simulink model "gm_Transformation_V12"  (R2018a)
settings: Solver=FixedStepDiscrete  StartTime=0.0  StopTime=10.0  RelTol=1e-3
InitFcn:
  | Ts_xadc = 0.1;
undefined symbols (not defined in the file or in its folder): T_25MHz, T_mech
libraries: hdlsllib x14, simulink x12, hdlmdlgenlib x5, simulink_need_slupdate x1
(part 2 of 4)

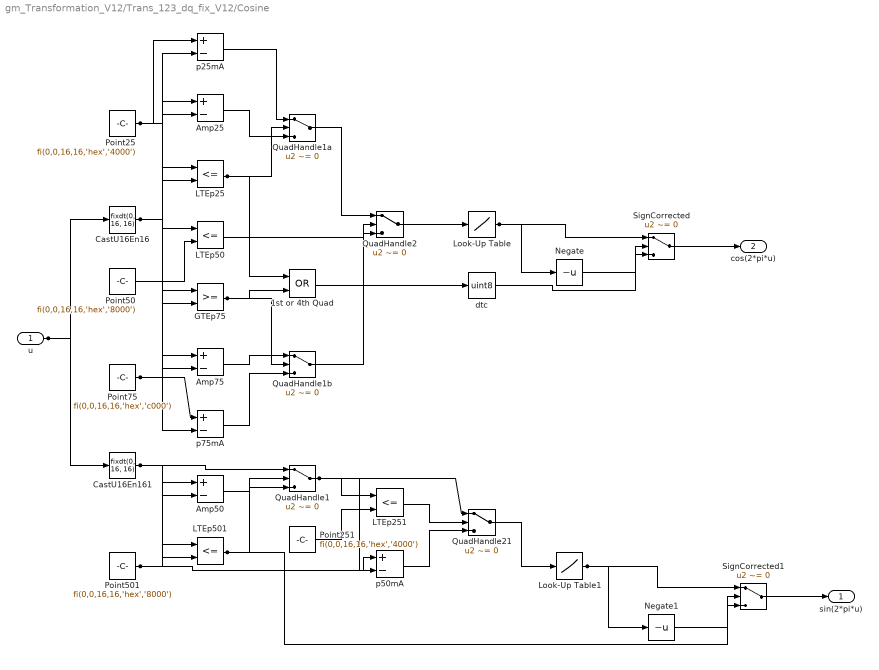
== system gm_Transformation_V12/Trans_123_dq_fix_V12/Cosine ==
  u : Inport  OutDataTypeStr=fixdt(1, 24, 20)  SampleTime=4e-08
  1st or 4th Quad : Logic  Operator=OR  AllPortsSameDT=off  OutDataTypeStr=boolean  SampleTime=4e-08
  Amp25 : Sum  Inputs=+-  AccumDataTypeStr=fixdt(1, 17, 16)  OutDataTypeStr=fixdt(1, 17, 16)  SampleTime=4e-08
  Amp50 : Sum  Inputs=+-  AccumDataTypeStr=fixdt(1, 17, 16)  OutDataTypeStr=fixdt(1, 17, 16)  SampleTime=4e-08
  Amp75 : Sum  Inputs=+-  AccumDataTypeStr=fixdt(1, 17, 16)  OutDataTypeStr=fixdt(1, 17, 16)  SampleTime=4e-08
  CastU16En16 : DataTypeConversion  OutDataTypeStr=fixdt(0, 16, 16)  SampleTime=4e-08
  CastU16En161 : DataTypeConversion  OutDataTypeStr=fixdt(0, 16, 16)  SampleTime=4e-08
  GTEp75 : RelationalOperator  OutDataTypeStr=boolean  SampleTime=4e-08  RndMeth=Nearest
  LTEp{25,50,251,501} (4 alike) : RelationalOperator  Operator=<=  OutDataTypeStr=boolean  SampleTime=4e-08  RndMeth=Nearest
  Look-Up Table : Lookup_n-D  NumberOfTableDimensions=1  BreakpointsForDimension1=[0 0.00048828125 0.0009765625 0.00146484375 0.001953125 0.00244140625 0.0029296875 0.00341796875 0.00390625 0.00439453125 0.0048828125 0.00537109375 0.005859375 0.00634765625 0.0068359375 0.00732421875 0.0078125 0.00830078125 0.0087890625 0.00927734375 0.009765625 0.01025390625 0.0107421875 0.01123046875 0.01171875 0.01220703125 0.0126953125 0.01318359375 0.013671875 0.01416015625 0.0146484375 0.01513671875 0.015625 0.01611328125 0.0166015625 0.01708984375 0.017578125 0.01806640625 0.0185546875 0.01904296875 0.01953125 0.02001953125 0.0205078125 0.02099609375 0.021484375 0.02197265625 0.0224609375 0.02294921875 0.0234375 0.02392578125 0.0244140625 0.02490234375 0.025390625 0.02587890625 0.0263671875 0.02685546875 0.02734375 0.02783203125 0.0283203125 0.02880859375 0.029296875 0.02978515625 0.0302734375 0.03076171875 0.03125 0.03173828125 0.0322265625 0.03271484375 0.033203125 0.03369140625 0.0341796875 0.03466796875 0.03515625 0.03564453125 0.0361328125 0.03662109375 0.037109375 0.03759765625 0.0380859375 0.03857421875 0.0390625 0.03955078125 0.0400390625 0.04052734375 0.041015625 0.04150390625 0.0419921875 0.04248046875 0.04296875 0.04345703125 0.0439453125 0.04443359375 0.044921875 0.04541015625 0.0458984375 0.04638671875 0.046875 0.04736328125 0.0478515625 0.04833984375 0.048828125 0.04931640625 0.0498046875 0.05029296875 0.05078125 0.05126953125 0.0517578125 0.05224609375 0.052734375 0.05322265625 0.0537109375 0.05419921875 0.0546875 0.05517578125 0.0556640625 0.05615234375 0.056640625 0.05712890625 0.0576171875 0.05810546875 0.05859375 0.05908203125 0.0595703125 0.06005859375 0.060546875 0.06103515625 0.0615234375 0.06201171875 0.0625 0.06298828125 0.0634765625 0.06396484375 0.064453125 0.06494140625 0.0654296875 0.06591796875 0.06640625 0.06689453125 0.0673828125 0.06787109375 0.068359375 0.06884765625 0.0693359375 0.06982421875 0.0703125 0.07080078125 0.0712890625 0.07177734375 0.072265625 0.07275390625 0.0732421875 0.07373046875 0.07421875 0.07470703125 0.0751953125 0.07568359375 0.076171875 0.07666015625 0.0771484375 0.07763671875 0.078125 0.07861328125 0.0791015625 0.07958984375 0.080078125 0.08056640625 0.0810546875 0.08154296875 0.08203125 0.08251953125 0.0830078125 0.08349609375 0.083984375 0.08447265625 0.0849609375 0.08544921875 0.0859375 0.08642578125 0.0869140625 0.08740234375 0.087890625 0.08837890625 0.0888671875 0.08935546875 0.08984375 0.09033203125 0.0908203125 0.09130859375 0.091796875 0.09228515625 0.0927734375 0.09326171875 0.09375 0.09423828125 0.0947265625 0.09521484375 0.095703125 0.09619140625 0.0966796875 0.09716796875 0.09765625 0.09814453125 0.0986328125 0.09912109375 0.099609375 0.10009765625 0.1005859375 0.10107421875 0.1015625 0.10205078125 0.1025390625 0.10302734375 0.103515625 0.10400390625 0.1044921875 0.10498046875 0.10546875 0.10595703125 0.1064453125 0.10693359375 0.107421875 0.10791015625 0.1083984375 0.10888671875 0.109375 0.10986328125 0.1103515625 0.11083984375 0.111328125 0.11181640625 0.1123046875 0.11279296875 0.11328125 0.11376953125 0.1142578125 0.11474609375 0.115234375 0.11572265625 0.1162109375 0.11669921875 0.1171875 0.11767578125 0.1181640625 0.11865234375 0.119140625 0.11962890625 0.1201171875 0.12060546875 0.12109375 0.12158203125 0.1220703125 0.12255859375 0.123046875 0.12353515625 0.1240234375 0.12451171875 0.125 0.12548828125 0.1259765625 0.12646484375 0.126953125 0.12744140625 0.1279296875 0.12841796875 0.12890625 0.12939453125 0.1298828125 0.13037109375 0.130859375 0.13134765625 0.1318359375 0.13232421875 0.1328125 0.13330078125 0.1337890625 0.13427734375 0.134765625 0.13525390625 0.1357421875 0.13623046875 0.13671875 0.13720703125 0.1376953125 0.13818359375 0.138671875 0.13916015625 0.1396484375 0.14013671875 0.140625 0.14111328125 0.1416015625 0.14208984375 0.142578125 0.14306640625 0.1435546875 0.14404296875 0.14453125 0.14501953125 0.1455078125 0.14599609375 0.146484375 0.14697265625 0.1474609375 0.14794921875 0.1484375 0.14892578125 0.1494140625 0.14990234375 ...(+2661 chars)]  Table="reshape([0;0.0030517578125;0.00616455078125;0.00921630859375;0.01226806640625;0.01531982421875;0.0184326171875;0.021484375;0.0245361328125;0.027587890625;0.03070068359375;0.03375244140625;0.03680419921875;0.03985595703125;0.04296875;0.0460205078125;0.049072265625;0.0521240234375;0.05517578125;0.05828857421875;0.06134033203125;0.06439208984375;0.06744384765625;0.07049560546875;0.07354736328125;0.07659912109375;0.0797119140625;0.082763671875;0.0858154296875;0.0888671875;0.0919189453125;0.094970703125;0.0980224609375;0.10107421875;0.1041259765625;0.107177734375;0.1102294921875;0.11328125;0.1163330078125;0.119384765625;0.1224365234375;0.12542724609375;0.12847900390625;0.13153076171875;0.13458251953125;0.13763427734375;0.14068603515625;0.1436767578125;0.146728515625;0.1497802734375;0.15277099609375;0.15582275390625;0.15887451171875;0.161865234375;0.1649169921875;0.16796875;0.17095947265625;0.17401123046875;0.177001953125;0.17999267578125;0.18304443359375;0.18603515625;0.1890869140625;0.19207763671875;0.195068359375;0.1981201171875;0.20111083984375;0.2041015625;0.20709228515625;0.2100830078125;0.213134765625;0.21612548828125;0.2191162109375;0.22210693359375;0.22509765625;0.22808837890625;0.2310791015625;0.23406982421875;0.23699951171875;0.239990234375;0.24298095703125;0.2459716796875;0.2489013671875;0.25189208984375;0.2548828125;0.2578125;0.26080322265625;0.26373291015625;0.2667236328125;0.2696533203125;0.27264404296875;0.27557373046875;0.27850341796875;0.281494140625;0.284423828125;0.287353515625;0.290283203125;0.293212890625;0.296142578125;0.299072265625;0.302001953125;0.304931640625;0.307861328125;0.310791015625;0.31365966796875;0.31658935546875;0.31951904296875;0.3223876953125;0.3253173828125;0.32818603515625;0.33111572265625;0.333984375;0.3369140625;0.33978271484375;0.3426513671875;0.34552001953125;0.348388671875;0.351318359375;0.35418701171875;0.3570556640625;0.35992431640625;0.36273193359375;0.3656005859375;0.36846923828125;0.371337890625;0.3741455078125;0.37701416015625;0.37982177734375;0.3826904296875;0.385498046875;0.38836669921875;0.39117431640625;0.39398193359375;0.39678955078125;0.39959716796875;0.40240478515625;0.40521240234375;0.40802001953125;0.41082763671875;0.41363525390625;0.41644287109375;0.419189453125;0.4219970703125;0.4248046875;0.42755126953125;0.4302978515625;0.43310546875;0.43585205078125;0.4385986328125;0.44134521484375;0.444091796875;0.44683837890625;0.4495849609375;0.45233154296875;0.455078125;0.45782470703125;0.46051025390625;0.4632568359375;0.46600341796875;0.46868896484375;0.47137451171875;0.47412109375;0.476806640625;0.4794921875;0.482177734375;0.48486328125;0.487548828125;0.490234375;0.492919921875;0.49554443359375;0.49822998046875;0.50091552734375;0.5035400390625;0.50616455078125;0.50885009765625;0.511474609375;0.51409912109375;0.5167236328125;0.51934814453125;0.52197265625;0.52459716796875;0.5272216796875;0.52978515625;0.53240966796875;0.53497314453125;0.53759765625;0.5401611328125;0.542724609375;0.54534912109375;0.54791259765625;0.55047607421875;0.55303955078125;0.5555419921875;0.55810546875;0.5606689453125;0.56317138671875;0.56573486328125;0.5682373046875;0.57080078125;0.57330322265625;0.5758056640625;0.57830810546875;0.580810546875;0.58331298828125;0.5858154296875;0.5882568359375;0.59075927734375;0.59326171875;0.595703125;0.59814453125;0.60064697265625;0.60308837890625;0.60552978515625;0.60797119140625;0.61041259765625;0.61279296875;0.615234375;0.61767578125;0.62005615234375;0.6224365234375;0.6248779296875;0.62725830078125;0.629638671875;0.63201904296875;0.6343994140625;0.63677978515625;0.63909912109375;0.6414794921875;0.64385986328125;0.64617919921875;0.64849853515625;0.65081787109375;0.6531982421875;0.655517578125;0.6578369140625;0.66009521484375;0.66241455078125;0.66473388671875;0.6669921875;0.6693115234375;0.67156982421875;0.673828125;0.67608642578125;0.6783447265625;0.68060302734375;0.682861328125;0.68505859375;0.68731689453125;0.68951416015625;0.6917724609375;0.6939697265625;0.6961669921875 ...(+4158 chars)])"  ExtrapMethod=Clip  SampleTime=4e-08  OutDataTypeStr=fixdt(1, 16, 14)  InputSameDT=on
  Look-Up Table1 : Lookup_n-D  NumberOfTableDimensions=1  BreakpointsForDimension1=[0 0.00048828125 0.0009765625 0.00146484375 0.001953125 0.00244140625 0.0029296875 0.00341796875 0.00390625 0.00439453125 0.0048828125 0.00537109375 0.005859375 0.00634765625 0.0068359375 0.00732421875 0.0078125 0.00830078125 0.0087890625 0.00927734375 0.009765625 0.01025390625 0.0107421875 0.01123046875 0.01171875 0.01220703125 0.0126953125 0.01318359375 0.013671875 0.01416015625 0.0146484375 0.01513671875 0.015625 0.01611328125 0.0166015625 0.01708984375 0.017578125 0.01806640625 0.0185546875 0.01904296875 0.01953125 0.02001953125 0.0205078125 0.02099609375 0.021484375 0.02197265625 0.0224609375 0.02294921875 0.0234375 0.02392578125 0.0244140625 0.02490234375 0.025390625 0.02587890625 0.0263671875 0.02685546875 0.02734375 0.02783203125 0.0283203125 0.02880859375 0.029296875 0.02978515625 0.0302734375 0.03076171875 0.03125 0.03173828125 0.0322265625 0.03271484375 0.033203125 0.03369140625 0.0341796875 0.03466796875 0.03515625 0.03564453125 0.0361328125 0.03662109375 0.037109375 0.03759765625 0.0380859375 0.03857421875 0.0390625 0.03955078125 0.0400390625 0.04052734375 0.041015625 0.04150390625 0.0419921875 0.04248046875 0.04296875 0.04345703125 0.0439453125 0.04443359375 0.044921875 0.04541015625 0.0458984375 0.04638671875 0.046875 0.04736328125 0.0478515625 0.04833984375 0.048828125 0.04931640625 0.0498046875 0.05029296875 0.05078125 0.05126953125 0.0517578125 0.05224609375 0.052734375 0.05322265625 0.0537109375 0.05419921875 0.0546875 0.05517578125 0.0556640625 0.05615234375 0.056640625 0.05712890625 0.0576171875 0.05810546875 0.05859375 0.05908203125 0.0595703125 0.06005859375 0.060546875 0.06103515625 0.0615234375 0.06201171875 0.0625 0.06298828125 0.0634765625 0.06396484375 0.064453125 0.06494140625 0.0654296875 0.06591796875 0.06640625 0.06689453125 0.0673828125 0.06787109375 0.068359375 0.06884765625 0.0693359375 0.06982421875 0.0703125 0.07080078125 0.0712890625 0.07177734375 0.072265625 0.07275390625 0.0732421875 0.07373046875 0.07421875 0.07470703125 0.0751953125 0.07568359375 0.076171875 0.07666015625 0.0771484375 0.07763671875 0.078125 0.07861328125 0.0791015625 0.07958984375 0.080078125 0.08056640625 0.0810546875 0.08154296875 0.08203125 0.08251953125 0.0830078125 0.08349609375 0.083984375 0.08447265625 0.0849609375 0.08544921875 0.0859375 0.08642578125 0.0869140625 0.08740234375 0.087890625 0.08837890625 0.0888671875 0.08935546875 0.08984375 0.09033203125 0.0908203125 0.09130859375 0.091796875 0.09228515625 0.0927734375 0.09326171875 0.09375 0.09423828125 0.0947265625 0.09521484375 0.095703125 0.09619140625 0.0966796875 0.09716796875 0.09765625 0.09814453125 0.0986328125 0.09912109375 0.099609375 0.10009765625 0.1005859375 0.10107421875 0.1015625 0.10205078125 0.1025390625 0.10302734375 0.103515625 0.10400390625 0.1044921875 0.10498046875 0.10546875 0.10595703125 0.1064453125 0.10693359375 0.107421875 0.10791015625 0.1083984375 0.10888671875 0.109375 0.10986328125 0.1103515625 0.11083984375 0.111328125 0.11181640625 0.1123046875 0.11279296875 0.11328125 0.11376953125 0.1142578125 0.11474609375 0.115234375 0.11572265625 0.1162109375 0.11669921875 0.1171875 0.11767578125 0.1181640625 0.11865234375 0.119140625 0.11962890625 0.1201171875 0.12060546875 0.12109375 0.12158203125 0.1220703125 0.12255859375 0.123046875 0.12353515625 0.1240234375 0.12451171875 0.125 0.12548828125 0.1259765625 0.12646484375 0.126953125 0.12744140625 0.1279296875 0.12841796875 0.12890625 0.12939453125 0.1298828125 0.13037109375 0.130859375 0.13134765625 0.1318359375 0.13232421875 0.1328125 0.13330078125 0.1337890625 0.13427734375 0.134765625 0.13525390625 0.1357421875 0.13623046875 0.13671875 0.13720703125 0.1376953125 0.13818359375 0.138671875 0.13916015625 0.1396484375 0.14013671875 0.140625 0.14111328125 0.1416015625 0.14208984375 0.142578125 0.14306640625 0.1435546875 0.14404296875 0.14453125 0.14501953125 0.1455078125 0.14599609375 0.146484375 0.14697265625 0.1474609375 0.14794921875 0.1484375 0.14892578125 0.1494140625 0.14990234375 ...(+2661 chars)]  Table="reshape([0;0.0030517578125;0.00616455078125;0.00921630859375;0.01226806640625;0.01531982421875;0.0184326171875;0.021484375;0.0245361328125;0.027587890625;0.03070068359375;0.03375244140625;0.03680419921875;0.03985595703125;0.04296875;0.0460205078125;0.049072265625;0.0521240234375;0.05517578125;0.05828857421875;0.06134033203125;0.06439208984375;0.06744384765625;0.07049560546875;0.07354736328125;0.07659912109375;0.0797119140625;0.082763671875;0.0858154296875;0.0888671875;0.0919189453125;0.094970703125;0.0980224609375;0.10107421875;0.1041259765625;0.107177734375;0.1102294921875;0.11328125;0.1163330078125;0.119384765625;0.1224365234375;0.12542724609375;0.12847900390625;0.13153076171875;0.13458251953125;0.13763427734375;0.14068603515625;0.1436767578125;0.146728515625;0.1497802734375;0.15277099609375;0.15582275390625;0.15887451171875;0.161865234375;0.1649169921875;0.16796875;0.17095947265625;0.17401123046875;0.177001953125;0.17999267578125;0.18304443359375;0.18603515625;0.1890869140625;0.19207763671875;0.195068359375;0.1981201171875;0.20111083984375;0.2041015625;0.20709228515625;0.2100830078125;0.213134765625;0.21612548828125;0.2191162109375;0.22210693359375;0.22509765625;0.22808837890625;0.2310791015625;0.23406982421875;0.23699951171875;0.239990234375;0.24298095703125;0.2459716796875;0.2489013671875;0.25189208984375;0.2548828125;0.2578125;0.26080322265625;0.26373291015625;0.2667236328125;0.2696533203125;0.27264404296875;0.27557373046875;0.27850341796875;0.281494140625;0.284423828125;0.287353515625;0.290283203125;0.293212890625;0.296142578125;0.299072265625;0.302001953125;0.304931640625;0.307861328125;0.310791015625;0.31365966796875;0.31658935546875;0.31951904296875;0.3223876953125;0.3253173828125;0.32818603515625;0.33111572265625;0.333984375;0.3369140625;0.33978271484375;0.3426513671875;0.34552001953125;0.348388671875;0.351318359375;0.35418701171875;0.3570556640625;0.35992431640625;0.36273193359375;0.3656005859375;0.36846923828125;0.371337890625;0.3741455078125;0.37701416015625;0.37982177734375;0.3826904296875;0.385498046875;0.38836669921875;0.39117431640625;0.39398193359375;0.39678955078125;0.39959716796875;0.40240478515625;0.40521240234375;0.40802001953125;0.41082763671875;0.41363525390625;0.41644287109375;0.419189453125;0.4219970703125;0.4248046875;0.42755126953125;0.4302978515625;0.43310546875;0.43585205078125;0.4385986328125;0.44134521484375;0.444091796875;0.44683837890625;0.4495849609375;0.45233154296875;0.455078125;0.45782470703125;0.46051025390625;0.4632568359375;0.46600341796875;0.46868896484375;0.47137451171875;0.47412109375;0.476806640625;0.4794921875;0.482177734375;0.48486328125;0.487548828125;0.490234375;0.492919921875;0.49554443359375;0.49822998046875;0.50091552734375;0.5035400390625;0.50616455078125;0.50885009765625;0.511474609375;0.51409912109375;0.5167236328125;0.51934814453125;0.52197265625;0.52459716796875;0.5272216796875;0.52978515625;0.53240966796875;0.53497314453125;0.53759765625;0.5401611328125;0.542724609375;0.54534912109375;0.54791259765625;0.55047607421875;0.55303955078125;0.5555419921875;0.55810546875;0.5606689453125;0.56317138671875;0.56573486328125;0.5682373046875;0.57080078125;0.57330322265625;0.5758056640625;0.57830810546875;0.580810546875;0.58331298828125;0.5858154296875;0.5882568359375;0.59075927734375;0.59326171875;0.595703125;0.59814453125;0.60064697265625;0.60308837890625;0.60552978515625;0.60797119140625;0.61041259765625;0.61279296875;0.615234375;0.61767578125;0.62005615234375;0.6224365234375;0.6248779296875;0.62725830078125;0.629638671875;0.63201904296875;0.6343994140625;0.63677978515625;0.63909912109375;0.6414794921875;0.64385986328125;0.64617919921875;0.64849853515625;0.65081787109375;0.6531982421875;0.655517578125;0.6578369140625;0.66009521484375;0.66241455078125;0.66473388671875;0.6669921875;0.6693115234375;0.67156982421875;0.673828125;0.67608642578125;0.6783447265625;0.68060302734375;0.682861328125;0.68505859375;0.68731689453125;0.68951416015625;0.6917724609375;0.6939697265625;0.6961669921875 ...(+4158 chars)])"  ExtrapMethod=Clip  SampleTime=4e-08  OutDataTypeStr=fixdt(1, 16, 14)  InputSameDT=on
  Negate : UnaryMinus  SampleTime=4e-08
  Negate1 : UnaryMinus  SampleTime=4e-08
  Point25 : Constant  Value=fi(0,0,16,16,'hex','4000')  OutDataTypeStr=fixdt(0, 16, 16)  SampleTime=-1
  Point251 : Constant  Value=fi(0,0,16,16,'hex','4000')  OutDataTypeStr=fixdt(0, 16, 16)  SampleTime=-1
  Point50 : Constant  Value=fi(0,0,16,16,'hex','8000')  OutDataTypeStr=fixdt(0, 16, 16)  SampleTime=-1
  Point501 : Constant  Value=fi(0,0,16,16,'hex','8000')  OutDataTypeStr=fixdt(0, 16, 16)  SampleTime=-1
  Point75 : Constant  Value=fi(0,0,16,16,'hex','c000')  OutDataTypeStr=fixdt(0, 16, 16)  SampleTime=-1
  QuadHandle1 : Switch  Criteria=u2 ~= 0  Threshold=double(0)  OutDataTypeStr=fixdt(1, 17, 16)  SampleTime=4e-08
  QuadHandle1a : Switch  Criteria=u2 ~= 0  Threshold=double(0)  OutDataTypeStr=fixdt(1, 17, 16)  SampleTime=4e-08
  QuadHandle1b : Switch  Criteria=u2 ~= 0  Threshold=double(0)  OutDataTypeStr=fixdt(1, 17, 16)  SampleTime=4e-08
  QuadHandle2 : Switch  Criteria=u2 ~= 0  Threshold=double(0)  OutDataTypeStr=fixdt(1, 17, 16)  SampleTime=4e-08
  QuadHandle21 : Switch  Criteria=u2 ~= 0  Threshold=double(0)  OutDataTypeStr=fixdt(1, 18, 16)  SampleTime=4e-08
  SignCorrected : Switch  Criteria=u2 ~= 0  Threshold=double(0)  OutDataTypeStr=fixdt(1, 16, 14)  SampleTime=4e-08
  SignCorrected1 : Switch  Criteria=u2 ~= 0  Threshold=double(0)  OutDataTypeStr=fixdt(1, 16, 14)  SampleTime=4e-08
  dtc : DataTypeConversion  OutDataTypeStr=uint8  SampleTime=4e-08
  p25mA : Sum  Inputs=+-  AccumDataTypeStr=fixdt(1, 17, 16)  OutDataTypeStr=fixdt(1, 17, 16)  SampleTime=4e-08
  p50mA : Sum  Inputs=+-  AccumDataTypeStr=fixdt(1, 18, 16)  OutDataTypeStr=fixdt(1, 18, 16)  SampleTime=4e-08
  p75mA : Sum  Inputs=+-  AccumDataTypeStr=fixdt(1, 17, 16)  OutDataTypeStr=fixdt(1, 17, 16)  SampleTime=4e-08
  sin(2*pi*u) : Outport
  cos(2*pi*u) : Outport  Port=2
  wires:
  Look-Up Table/1 -> SignCorrected/1, Negate/1
  dtc/1 -> SignCorrected/2
  Amp25/1 -> QuadHandle1a/3
  Amp75/1 -> QuadHandle1b/1
  CastU16En16/1 -> p75mA/2, p25mA/2, LTEp50/1, LTEp25/1, GTEp75/1, Amp75/1, Amp25/1
  GTEp75/1 -> QuadHandle1b/2, 1st or 4th Quad/2
  LTEp25/1 -> QuadHandle1a/2, 1st or 4th Quad/1
  LTEp50/1 -> QuadHandle2/2
  Negate/1 -> SignCorrected/3
  Point25/1 -> p25mA/1, LTEp25/2, Amp25/2
  Point50/1 -> LTEp50/2
  Point75/1 -> p75mA/1, GTEp75/2, Amp75/2
  QuadHandle1a/1 -> QuadHandle2/1
  QuadHandle1b/1 -> QuadHandle2/3
  QuadHandle2/1 -> Look-Up Table/1
  SignCorrected/1 -> cos(2*pi*u)/1
  p25mA/1 -> QuadHandle1a/1
  p75mA/1 -> QuadHandle1b/3
  Look-Up Table1/1 -> SignCorrected1/1, Negate1/1
  Amp50/1 -> QuadHandle1/3
  CastU16En161/1 -> QuadHandle1/1, LTEp501/1, Amp50/1
  LTEp251/1 -> QuadHandle21/2
  LTEp501/1 -> SignCorrected1/2, QuadHandle1/2
  Negate1/1 -> SignCorrected1/3
  Point251/1 -> LTEp251/2
  Point501/1 -> p50mA/1, LTEp501/2, Amp50/2
  QuadHandle1/1 -> p50mA/2, QuadHandle21/1, LTEp251/1
  QuadHandle21/1 -> Look-Up Table1/1
  SignCorrected1/1 -> sin(2*pi*u)/1
  p50mA/1 -> QuadHandle21/3
  1st or 4th Quad/1 -> dtc/1
  u/1 -> CastU16En161/1, CastU16En16/1

== system gm_Transformation_V12/xadc/xadc_plant ==
  Addr : Inport
  V : Inport  Port=2
  Vaux : Inport  Port=3
  AuxChan : Subsystem
  Bit Slice : hdlsllib/Logic and Bit Operations/Bit Slice  lidx=3  ridx=0
  Bit Slice1 : hdlsllib/Logic and Bit Operations/Bit Slice  lidx=4  ridx=4
  IntChan : Subsystem
  Switch : Switch  Criteria=u2 ~= 0
  Data : Outport
  wires:
  AuxChan/1(Aux_ADC) -> Switch/1
  IntChan/1(Int_ADC) -> Switch/3
  Bit Slice1/1 -> Switch/2
  Switch/1 -> Data/1
  V/1 -> IntChan/2(V)
  Vaux/1 -> AuxChan/2(Vaux)
  Bit Slice/1 -> AuxChan/1(Addr), IntChan/1(Addr)
  Addr/1 -> Bit Slice/1, Bit Slice1/1

== system gm_Transformation_V12/DUT_V5/UnitConversion/ExtAmpConvert1 ==
  Raw : Inport
  Conv_Factor : Inport  Port=2
  Product : Product  OutDataTypeStr=fixdt(1,16,11)
  Amp : Outport
  wires:
  Conv_Factor/1 -> Product/2
  Product/1 -> Amp/1
  Raw/1 -> Product/1

== system gm_Transformation_V12/DUT_V5/UnitConversion/ExtAmpConvert2 ==
  Raw : Inport
  Conv_Factor : Inport  Port=2
  Product : Product  OutDataTypeStr=fixdt(1,16,11)
  Amp : Outport
  wires:
  Conv_Factor/1 -> Product/2
  Product/1 -> Amp/1
  Raw/1 -> Product/1

== system gm_Transformation_V12/DUT_V5/UnitConversion/ExtAmpConvert3 ==
  Raw : Inport
  Conv_Factor : Inport  Port=2
  Product : Product  OutDataTypeStr=fixdt(1,16,11)
  Amp : Outport
  wires:
  Conv_Factor/1 -> Product/2
  Product/1 -> Amp/1
  Raw/1 -> Product/1

== system gm_Transformation_V12/DUT_V5/UnitConversion/ExtVoltConvert1 ==
  Raw : Inport
  Gain : Gain  Gain=fi(1/4096)  OutMin=0  OutMax=1  OutDataTypeStr=fixdt(0,16)
  Volts : Outport
  wires:
  Gain/1 -> Volts/1
  Raw/1 -> Gain/1

== system gm_Transformation_V12/DUT_V5/UnitConversion/ExtVoltConvert2 ==
  Raw : Inport
  Gain : Gain  Gain=fi(1/4096)  OutMin=0  OutMax=1  OutDataTypeStr=fixdt(0,16)
  Volts : Outport
  wires:
  Raw/1 -> Gain/1
  Gain/1 -> Volts/1

== system gm_Transformation_V12/DUT_V5/UnitConversion/ExtVoltConvert3 ==
  Raw : Inport
  Gain : Gain  Gain=fi(1/4096)  OutMin=0  OutMax=1  OutDataTypeStr=fixdt(0,16)
  Volts : Outport
  wires:
  Gain/1 -> Volts/1
  Raw/1 -> Gain/1

== system gm_Transformation_V12/DUT_V5/UnitConversion/IntVoltConvert ==
  Raw : Inport
  Gain : Gain  Gain=fi(3/4096)  OutMin=0  OutMax=3  OutDataTypeStr=fixdt(0,16)
  Volts : Outport
  wires:
  Gain/1 -> Volts/1
  Raw/1 -> Gain/1

== system gm_Transformation_V12/DUT_V5/UnitConversion/TempConvert ==
  Raw : Inport
  Add : Sum  Inputs=+-
  Constant : Constant  Value=273.15  OutDataTypeStr=fixdt(0,15)  SampleTime=-1
  Gain : Gain  Gain=fi(503.975/4096)  OutMin=0  OutMax=503.975  OutDataTypeStr=fixdt(0,15)
  DegC : Outport
  wires:
  Raw/1 -> Gain/1
  Add/1 -> DegC/1
  Constant/1 -> Add/2
  Gain/1 -> Add/1

== system gm_Transformation_V12/xadc/xadc_plant/AuxChan ==
  Addr : Inport
  Vaux : Inport  Port=2
  Demux : Demux  Outputs=16
  ExtVoltPlant19 : Subsystem
  Multiport Switch1 : MultiPortSwitch  DataPortOrder=Zero-based contiguous  Inputs=16  DiagnosticForDefault=None  zeroidx=on
  Aux_ADC : Outport
  wires:
  Demux/16 -> Multiport Switch1/17
  Addr/1 -> Multiport Switch1/1
  Demux/15 -> Multiport Switch1/16
  Multiport Switch1/1 -> Aux_ADC/1
  Demux/9 -> Multiport Switch1/10
  Vaux/1 -> ExtVoltPlant19/1(Volts)
  Demux/7 -> Multiport Switch1/8
  Demux/5 -> Multiport Switch1/6
  Demux/13 -> Multiport Switch1/14
  Demux/11 -> Multiport Switch1/12
  Demux/10 -> Multiport Switch1/11
  Demux/4 -> Multiport Switch1/5
  Demux/14 -> Multiport Switch1/15
  Demux/6 -> Multiport Switch1/7
  Demux/12 -> Multiport Switch1/13
  Demux/8 -> Multiport Switch1/9
  Demux/2 -> Multiport Switch1/3
  Demux/3 -> Multiport Switch1/4
  Demux/1 -> Multiport Switch1/2
  ExtVoltPlant19/1(Raw_ADC) -> Demux/1

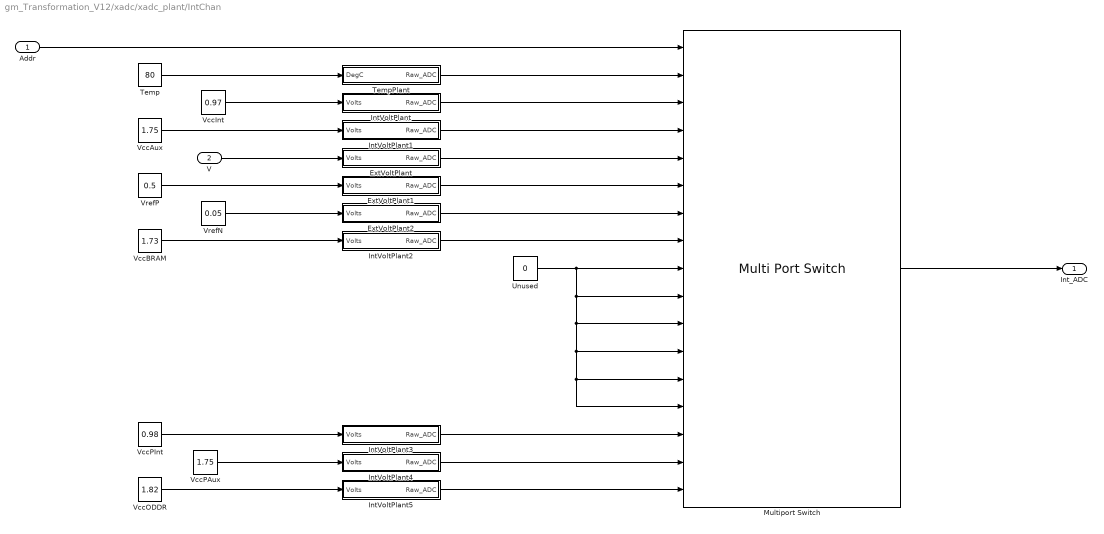
== system gm_Transformation_V12/xadc/xadc_plant/IntChan ==
  Addr : Inport
  V : Inport  Port=2
  ExtVoltPlant : Subsystem
  ExtVoltPlant1 : Subsystem
  ExtVoltPlant2 : Subsystem
  IntVoltPlant : Subsystem
  IntVoltPlant1 : Subsystem
  IntVoltPlant2 : Subsystem
  IntVoltPlant3 : Subsystem
  IntVoltPlant4 : Subsystem
  IntVoltPlant5 : Subsystem
  Multiport Switch : MultiPortSwitch  DataPortOrder=Zero-based contiguous  Inputs=16  DiagnosticForDefault=None  zeroidx=on
  Temp : Constant  Value=80  SampleTime=-1
  TempPlant : Subsystem
  Unused : Constant  Value=0  OutDataTypeStr=Inherit: Inherit via back propagation  SampleTime=-1
  VccAux : Constant  Value=1.75  SampleTime=-1
  VccBRAM : Constant  Value=1.73  SampleTime=-1
  VccInt : Constant  Value=0.97  SampleTime=-1
  VccODDR : Constant  Value=1.82  SampleTime=-1
  VccPAux : Constant  Value=1.75  SampleTime=-1
  VccPInt : Constant  Value=0.98  SampleTime=-1
  VrefN : Constant  Value=0.05  SampleTime=-1
  VrefP : Constant  Value=0.5  SampleTime=-1
  Int_ADC : Outport
  wires:
  VrefP/1 -> ExtVoltPlant1/1(Volts)
  ExtVoltPlant1/1(Raw_ADC) -> Multiport Switch/6
  IntVoltPlant1/1(Raw_ADC) -> Multiport Switch/4
  Unused/1 -> Multiport Switch/10, Multiport Switch/11, Multiport Switch/12, Multiport Switch/13, Multiport Switch/14, Multiport Switch/9
  IntVoltPlant/1(Raw_ADC) -> Multiport Switch/3
  Multiport Switch/1 -> Int_ADC/1
  Addr/1 -> Multiport Switch/1
  IntVoltPlant3/1(Raw_ADC) -> Multiport Switch/15
  VccBRAM/1 -> IntVoltPlant2/1(Volts)
  VccAux/1 -> IntVoltPlant1/1(Volts)
  VccPInt/1 -> IntVoltPlant3/1(Volts)
  VccPAux/1 -> IntVoltPlant4/1(Volts)
  ExtVoltPlant/1(Raw_ADC) -> Multiport Switch/5
  Temp/1 -> TempPlant/1(DegC)
  IntVoltPlant4/1(Raw_ADC) -> Multiport Switch/16
  VccInt/1 -> IntVoltPlant/1(Volts)
  TempPlant/1(Raw_ADC) -> Multiport Switch/2
  ExtVoltPlant2/1(Raw_ADC) -> Multiport Switch/7
  V/1 -> ExtVoltPlant/1(Volts)
  IntVoltPlant5/1(Raw_ADC) -> Multiport Switch/17
  VrefN/1 -> ExtVoltPlant2/1(Volts)
  VccODDR/1 -> IntVoltPlant5/1(Volts)
  IntVoltPlant2/1(Raw_ADC) -> Multiport Switch/8

== system gm_Transformation_V12/xadc/xadc_plant/AuxChan/ExtVoltPlant19 ==
  Volts : Inport
  Bit Concat : hdlsllib/Logic and Bit Operations/Bit Concat  numInputs=2
      settings: SourceProductName=HDL Coder  SourceProductBaseCode=HD
  Data Type Conversion : DataTypeConversion  OutDataTypeStr=fixdt(0,12,0)
  Gain : Gain  Gain=4096
  LSB : Constant  Value=fi(0,0,4,0)  SampleTime=-1
  Raw_ADC : Outport
  wires:
  Gain/1 -> Data Type Conversion/1
  Volts/1 -> Gain/1
  Data Type Conversion/1 -> Bit Concat/1
  LSB/1 -> Bit Concat/2
  Bit Concat/1 -> Raw_ADC/1

== system gm_Transformation_V12/xadc/xadc_plant/IntChan/ExtVoltPlant ==
  Volts : Inport
  Bit Concat : hdlsllib/Logic and Bit Operations/Bit Concat  numInputs=2
      settings: SourceProductName=HDL Coder  SourceProductBaseCode=HD
  Data Type Conversion : DataTypeConversion  OutDataTypeStr=fixdt(0,12,0)
  Gain : Gain  Gain=4096
  LSB : Constant  Value=fi(0,0,4,0)  SampleTime=-1
  Raw_ADC : Outport
  wires:
  Gain/1 -> Data Type Conversion/1
  Volts/1 -> Gain/1
  Data Type Conversion/1 -> Bit Concat/1
  LSB/1 -> Bit Concat/2
  Bit Concat/1 -> Raw_ADC/1

== system gm_Transformation_V12/xadc/xadc_plant/IntChan/ExtVoltPlant1 ==
  Volts : Inport
  Bit Concat : hdlsllib/Logic and Bit Operations/Bit Concat  numInputs=2
      settings: SourceProductName=HDL Coder  SourceProductBaseCode=HD
  Data Type Conversion : DataTypeConversion  OutDataTypeStr=fixdt(0,12,0)
  Gain : Gain  Gain=4096
  LSB : Constant  Value=fi(0,0,4,0)  SampleTime=-1
  Raw_ADC : Outport
  wires:
  Bit Concat/1 -> Raw_ADC/1
  LSB/1 -> Bit Concat/2
  Data Type Conversion/1 -> Bit Concat/1
  Volts/1 -> Gain/1
  Gain/1 -> Data Type Conversion/1

== system gm_Transformation_V12/xadc/xadc_plant/IntChan/ExtVoltPlant2 ==
  Volts : Inport
  Bit Concat : hdlsllib/Logic and Bit Operations/Bit Concat  numInputs=2
      settings: SourceProductName=HDL Coder  SourceProductBaseCode=HD
  Data Type Conversion : DataTypeConversion  OutDataTypeStr=fixdt(0,12,0)
  Gain : Gain  Gain=4096
  LSB : Constant  Value=fi(0,0,4,0)  SampleTime=-1
  Raw_ADC : Outport
  wires:
  Gain/1 -> Data Type Conversion/1
  Volts/1 -> Gain/1
  Data Type Conversion/1 -> Bit Concat/1
  LSB/1 -> Bit Concat/2
  Bit Concat/1 -> Raw_ADC/1

== system gm_Transformation_V12/xadc/xadc_plant/IntChan/IntVoltPlant ==
  Volts : Inport
  Bit Concat : hdlsllib/Logic and Bit Operations/Bit Concat  numInputs=2
      settings: SourceProductName=HDL Coder  SourceProductBaseCode=HD
  Data Type Conversion : DataTypeConversion  OutDataTypeStr=fixdt(0,12,0)
  Gain : Gain  Gain=4096/3
  LSB : Constant  Value=fi(0,0,4,0)  SampleTime=-1
  Raw_ADC : Outport
  wires:
  Bit Concat/1 -> Raw_ADC/1
  LSB/1 -> Bit Concat/2
  Data Type Conversion/1 -> Bit Concat/1
  Volts/1 -> Gain/1
  Gain/1 -> Data Type Conversion/1

== system gm_Transformation_V12/xadc/xadc_plant/IntChan/IntVoltPlant1 ==
  Volts : Inport
  Bit Concat : hdlsllib/Logic and Bit Operations/Bit Concat  numInputs=2
      settings: SourceProductName=HDL Coder  SourceProductBaseCode=HD
  Data Type Conversion : DataTypeConversion  OutDataTypeStr=fixdt(0,12,0)
  Gain : Gain  Gain=4096/3
  LSB : Constant  Value=fi(0,0,4,0)  SampleTime=-1
  Raw_ADC : Outport
  wires:
  Gain/1 -> Data Type Conversion/1
  Volts/1 -> Gain/1
  Data Type Conversion/1 -> Bit Concat/1
  LSB/1 -> Bit Concat/2
  Bit Concat/1 -> Raw_ADC/1

== system gm_Transformation_V12/xadc/xadc_plant/IntChan/IntVoltPlant2 ==
  Volts : Inport
  Bit Concat : hdlsllib/Logic and Bit Operations/Bit Concat  numInputs=2
      settings: SourceProductName=HDL Coder  SourceProductBaseCode=HD
  Data Type Conversion : DataTypeConversion  OutDataTypeStr=fixdt(0,12,0)
  Gain : Gain  Gain=4096/3
  LSB : Constant  Value=fi(0,0,4,0)  SampleTime=-1
  Raw_ADC : Outport
  wires:
  Bit Concat/1 -> Raw_ADC/1
  LSB/1 -> Bit Concat/2
  Data Type Conversion/1 -> Bit Concat/1
  Volts/1 -> Gain/1
  Gain/1 -> Data Type Conversion/1

== system gm_Transformation_V12/xadc/xadc_plant/IntChan/IntVoltPlant3 ==
  Volts : Inport
  Bit Concat : hdlsllib/Logic and Bit Operations/Bit Concat  numInputs=2
      settings: SourceProductName=HDL Coder  SourceProductBaseCode=HD
  Data Type Conversion : DataTypeConversion  OutDataTypeStr=fixdt(0,12,0)
  Gain : Gain  Gain=4096/3
  LSB : Constant  Value=fi(0,0,4,0)  SampleTime=-1
  Raw_ADC : Outport
  wires:
  Gain/1 -> Data Type Conversion/1
  Volts/1 -> Gain/1
  Data Type Conversion/1 -> Bit Concat/1
  LSB/1 -> Bit Concat/2
  Bit Concat/1 -> Raw_ADC/1

== system gm_Transformation_V12/xadc/xadc_plant/IntChan/IntVoltPlant4 ==
  Volts : Inport
  Bit Concat : hdlsllib/Logic and Bit Operations/Bit Concat  numInputs=2
      settings: SourceProductName=HDL Coder  SourceProductBaseCode=HD
  Data Type Conversion : DataTypeConversion  OutDataTypeStr=fixdt(0,12,0)
  Gain : Gain  Gain=4096/3
  LSB : Constant  Value=fi(0,0,4,0)  SampleTime=-1
  Raw_ADC : Outport
  wires:
  Bit Concat/1 -> Raw_ADC/1
  LSB/1 -> Bit Concat/2
  Data Type Conversion/1 -> Bit Concat/1
  Volts/1 -> Gain/1
  Gain/1 -> Data Type Conversion/1

== system gm_Transformation_V12/xadc/xadc_plant/IntChan/IntVoltPlant5 ==
  Volts : Inport
  Bit Concat : hdlsllib/Logic and Bit Operations/Bit Concat  numInputs=2
      settings: SourceProductName=HDL Coder  SourceProductBaseCode=HD
  Data Type Conversion : DataTypeConversion  OutDataTypeStr=fixdt(0,12,0)
  Gain : Gain  Gain=4096/3
  LSB : Constant  Value=fi(0,0,4,0)  SampleTime=-1
  Raw_ADC : Outport
  wires:
  Gain/1 -> Data Type Conversion/1
  Volts/1 -> Gain/1
  Data Type Conversion/1 -> Bit Concat/1
  LSB/1 -> Bit Concat/2
  Bit Concat/1 -> Raw_ADC/1

== system gm_Transformation_V12/xadc/xadc_plant/IntChan/TempPlant ==
  DegC : Inport
  Add : Sum
  Bit Concat : hdlsllib/Logic and Bit Operations/Bit Concat  numInputs=2
      settings: SourceProductName=HDL Coder  SourceProductBaseCode=HD
  Data Type Conversion : DataTypeConversion  OutDataTypeStr=fixdt(0,12,0)
  Gain : Gain  Gain=4096/503.975
  LSB : Constant  Value=fi(0,0,4,0)  SampleTime=-1
  Offset : Constant  Value=273.15  SampleTime=-1
  Raw_ADC : Outport
  wires:
  Bit Concat/1 -> Raw_ADC/1
  Gain/1 -> Data Type Conversion/1
  LSB/1 -> Bit Concat/2
  Data Type Conversion/1 -> Bit Concat/1
  Add/1 -> Gain/1
  DegC/1 -> Add/1
  Offset/1 -> Add/2
